simulink subsystem "Unpack_Param"  (R2025b)
settings: Solver=VariableStepAuto  StartTime=0.0  StopTime=10.0  RelTol=1e-3
libraries: simulink x1, etargetslib x1
settings Model: DataDictionary=Data_Param.sldd  EnableAccessToBaseWorkspace=off  Creator=damerius  LastModifiedBy=damerius

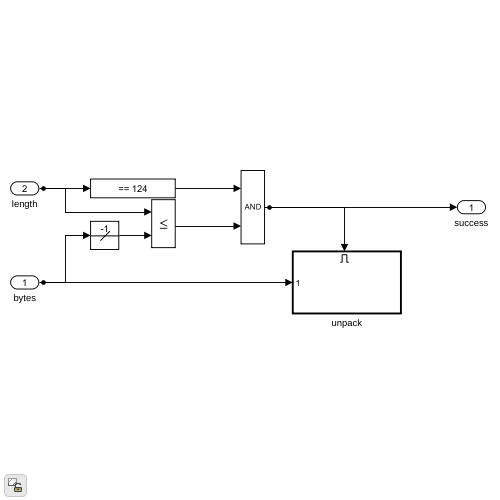
[thumbnail: Simulink's stored preview of the top-level diagram]
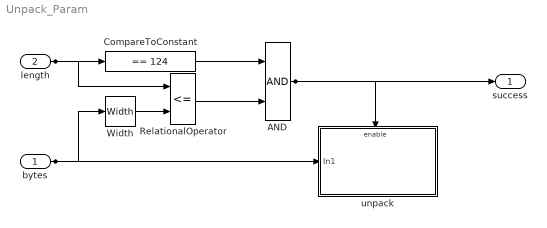
== system Unpack_Param ==
  bytes : Inport  OutDataTypeStr=uint8
  length : Inport  Port=2  OutDataTypeStr=uint32  PortDimensions=1
  AND : Logic  AllPortsSameDT=off  OutDataTypeStr=boolean
  CompareToConstant : simulink/Logic and Bit Operations/Compare To Constant  relop===  const=124  OutDataTypeStr=boolean
  RelationalOperator : RelationalOperator  Operator=<=  OutDataTypeStr=boolean  RndMeth=Simplest  InputSameDT=off
  Width : Width  DataType=uint32
  unpack : Subsystem  TreatAsAtomicUnit=on
  success : Outport  OutDataTypeStr=boolean  PortDimensions=1
  wires:
  length/1 -> RelationalOperator/1, CompareToConstant/1
  bytes/1 -> Width/1, unpack/1(In1)
  Width/1 -> RelationalOperator/2
  CompareToConstant/1 -> AND/1
  RelationalOperator/1 -> AND/2
  AND/1 -> unpack/Enable, success/1

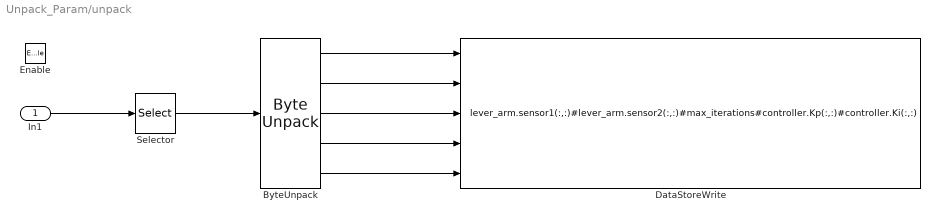
== system Unpack_Param/unpack ==
  In1 : Inport
  Enable : EnablePort
  ByteUnpack : etargetslib/Byte Unpack  dimensions={[3 1],[3 1],1,[3 3],[3 3]}  datatypes={'double','double','int32','single','single'}  byteAlign=1
      settings: LibrarySourceBlock=embeddedtargetslib/Host Communication/Byte Unpack
  DataStoreWrite : DataStoreWrite  DataStoreName=datastoreParam  DataStoreElements=lever_arm.sensor1(:,:)#lever_arm.sensor2(:,:)#max_iterations#controller.Kp(:,:)#controller.Ki(:,:)  IndexOptions=Index vector (dialog)  Indices=1  OutputSizes=1
  Selector : Selector  IndexOptions=Index vector (dialog)  Indices=1:124  OutputSizes=1
  wires:
  In1/1 -> Selector/1
  Selector/1 -> ByteUnpack/1
  ByteUnpack/1 -> DataStoreWrite/1
  ByteUnpack/2 -> DataStoreWrite/2
  ByteUnpack/3 -> DataStoreWrite/3
  ByteUnpack/4 -> DataStoreWrite/4
  ByteUnpack/5 -> DataStoreWrite/5
